simulink model "VGWEC_Model"  (R2022a)
settings: Solver=ode3  StartTime=0.0  StopTime=tSim  FixedStep=dt  RelTol=1e-3
undefined symbols (not defined in the file): amp_Wave, hydroCoeff, hydroVCoeff, theta0, w_Wave
settings Model: Creator=tdemonte  LastModifiedBy=tdemonte

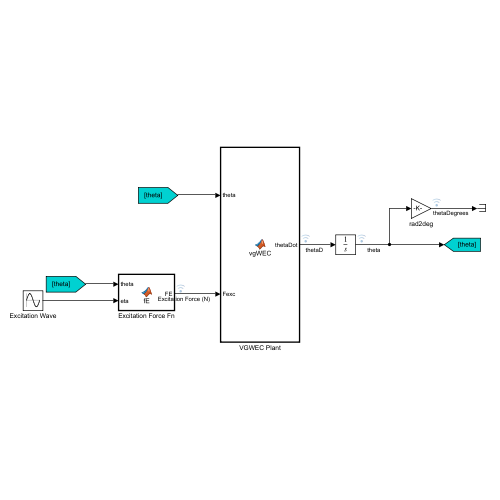
[thumbnail: Simulink's stored preview of the top-level diagram]
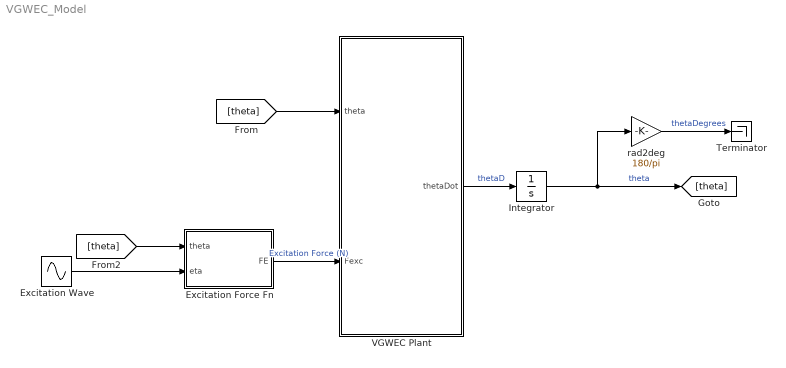
== system VGWEC_Model ==
  Excitation Force Fn : MATLAB Function  TreatAsAtomicUnit=on
  Excitation Wave : Sin  Amplitude=amp_Wave  Frequency=w_Wave  SampleTime=0
  Integrator : Integrator  InitialCondition=theta0
  Terminator : Terminator
  VGWEC Plant : MATLAB Function  TreatAsAtomicUnit=on
  rad2deg : Gain  Gain=180/pi
  wires:
  VGWEC Plant/1(thetaDot) -> Integrator/1  "thetaD"
  Integrator/1 -> rad2deg/1, [theta]  "theta"
  [theta] -> VGWEC Plant/1(theta)
  Excitation Force Fn/1(FE) -> VGWEC Plant/2(Fexc)  "Excitation Force (N)"
  Excitation Wave/1 -> Excitation Force Fn/2(eta)
  [theta] -> Excitation Force Fn/1(theta)
  rad2deg/1 -> Terminator/1  "thetaDegrees"

== matlab function VGWEC_Model/VGWEC Plant ==
  data: theta input size=2; thetaDot output size=[1 2]; Fexc input size=1; hydroVCoeff parameter; hydroCoeff parameter; w_Wave parameter
function thetaDot = vgWEC(theta, Fexc, hydroVCoeff, hydroCoeff, w_Wave)

% Declare the plant as an extrinsic function
%coder.extrinsic('vgWecPlant');

thetaDot = vgWecPlant(theta,w_Wave,hydroCoeff,hydroVCoeff, Fexc);

== matlab function VGWEC_Model/Excitation Force Fn ==
  data: theta input size=[1 2]; FE output double size=1; eta input size=1; hydroCoeff parameter; hydroVCoeff parameter; w_Wave parameter
function FE = fE(theta,eta,hydroCoeff, hydroVCoeff, w_Wave)

% Declare the excitation force function as an extrinsic function
%coder.extrinsic('fExc');

FE = fExc(theta, eta, w_Wave,hydroVCoeff,hydroCoeff);
